simulink model "test_tx_bf"  (R2020a)
settings: Solver=VariableStepAuto  StartTime=0.0  StopTime=180*system.step  RelTol=1e-3
undefined symbols (not defined in the file or in its folder): physconst, system
libraries: simulink x2, phasedtxrxlib x1, phasedbflib x1
settings Model: Creator=jose_  LastModifiedBy=jose_

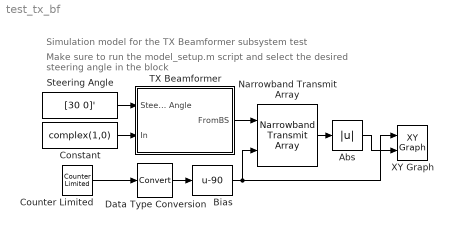
== system test_tx_bf ==
  note: Make sure to run the model_setup.m script and select the desired steering angle in the block
  note: Simulation model for the TX Beamformer subsystem test
  Abs : Abs
  Bias : Bias  Bias=-90
  Constant : Constant  Value=complex(1,0)
  Counter Limited : simulink/Sources/Counter Limited  uplimit=359  tsamp=system.step
  Data Type Conversion : DataTypeConversion
  Narrowband Transmit Array : phasedtxrxlib/Narrowband Transmit Array  PropagationSpeed=physconst( 'LightSpeed' )  OperatingFrequency=system.freq  CombineRadiatedSignals=on  SensorGainMeasure=dB  Polarization=None  WeightsInputPort=off  SimulateUsing=Code generation  Sensor=AntennaArray
      settings: SourceProductBaseCode=AR
  Steering Angle : Constant  Value=[30 0]'
  TX Beamformer : Subsystem
      mask Display: image('$imagefile'); % Use "Edit Image" on toolstrip to change.
  XY Graph : simulink/Sinks/XY Graph  xmin=-90  xmax=90  ymin=0  ymax=1.5  st=-1
  wires:
  Constant/1 -> TX Beamformer/2(In)
  Steering Angle/1 -> TX Beamformer/1(Steering Angle)
  Counter Limited/1 -> Data Type Conversion/1
  Data Type Conversion/1 -> Bias/1
  Bias/1 -> XY Graph/1, Narrowband Transmit Array/2
  TX Beamformer/1(FromBS) -> Narrowband Transmit Array/1
  Narrowband Transmit Array/1 -> Abs/1
  Abs/1 -> XY Graph/2

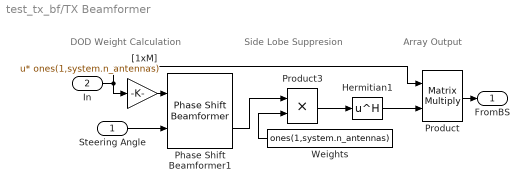
== system test_tx_bf/TX Beamformer ==
  note: Array Output
  note: Side Lobe Suppresion
  note: DOD Weight Calculation
  Steering Angle : Inport
  In : Inport  Port=2
  Hermitian1 : Math  Operator=hermitian  SaturateOnIntegerOverflow=on
  Phase Shift Beamformer1 : phasedbflib/Phase Shift Beamformer  PropagationSpeed=physconst( 'LightSpeed' )  OperatingFrequency=system.freq  DirectionSource=Input port  Direction=[ 0; 0 ]  NumPhaseShifterBits=0  WeightsNormalization=Preserve power  WeightsOutputPort=on  SimulateUsing=Code generation  SensorArray=AntennaArray
      settings: SourceProductBaseCode=AR
  Product : Product  Multiplication=Matrix(*)
  Product3 : Product
  Weights : Constant  Value=ones(1,system.n_antennas)  SampleTime=system.step
  "[1xM]" : Gain  Gain=ones(1,system.n_antennas)  Multiplication=Matrix(u*K)
  FromBS : Outport
  wires:
  Weights/1 -> Product3/2
  Phase Shift Beamformer1/2 -> Product3/1
  Steering Angle/1 -> Phase Shift Beamformer1/2
  Hermitian1/1 -> Product/2
  Product3/1 -> Hermitian1/1
  Product/1 -> FromBS/1
  In/1 -> "[1xM]"/1, Product/1
  "[1xM]"/1 -> Phase Shift Beamformer1/1
